simulink model "PMSM_Sinusoidal"  (R2023a)
settings: Solver=ode23t  StartTime=0.0  StopTime=5e-3  MaxStep=5e-8  RelTol=1e-5
libraries: fl_lib x4, SLSS x4, simulink_extras x1, PMSM x1, nesl_utility x1
settings Model: Creator=Szalay  LastModifiedBy=Szalay
settings SolverCC: AlgebraicLoopSolver=TrustRegion
settings DebuggingCC: UnconnectedInputMsg=warning  UnconnectedOutputMsg=warning  UnconnectedLineMsg=warning
settings ModelReferenceCC: EnableRefExpFcnMdlSchedulingChecks=on
settings RTWCC: DLArmComputeVersion=19.05
settings SimscapeCC: SimscapeLogType=all  SimscapeLogLimitData=off

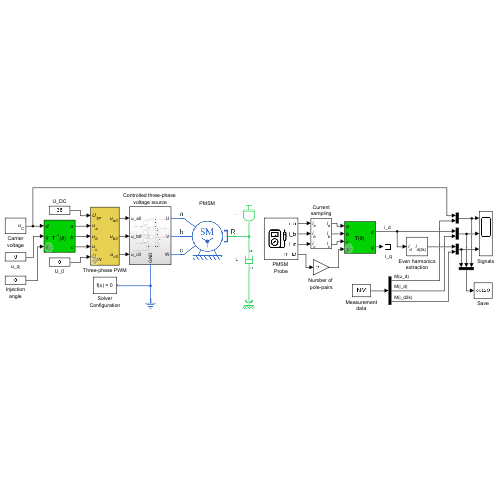
[thumbnail: Simulink's stored preview of the top-level diagram]
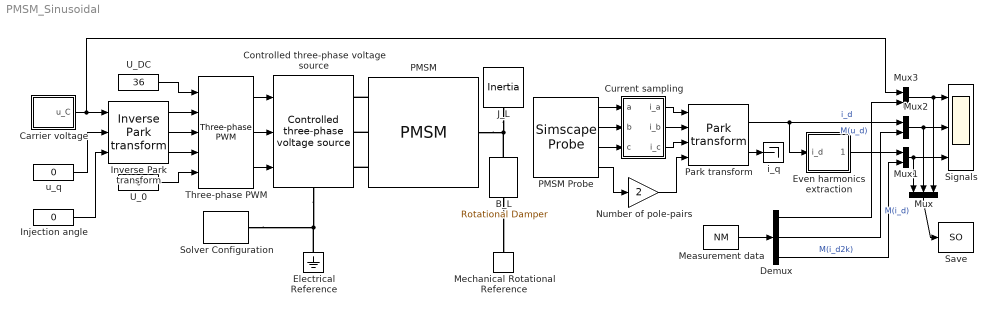
== system PMSM_Sinusoidal ==
  B_L : fl_lib/Mechanical/Rotational Elements/Rotational Damper  D=0.001 N*m*s/rad  w_specify=off  w_priority=None  w=0 rad/s  w_nominal_specify=off  w_nominal_unit=rad/s  w_nominal_value=1  t_specify=off  t_priority=None  t=0 N*m  t_nominal_specify=off  t_nominal_unit=N*m  t_nominal_value=1
  Carrier voltage : Subsystem
      mask Display: port_label('output', 1, '\itu_C', 'texmode', 'on');
  Controlled three-phase voltage source : SLSS/Power electronics/Controlled three-phase voltage source  SystemSampleTime=-1  VariantActivationTime=update diagram  Latency=0  AutoFrameSizeCalculation=off
      settings: PortSchema="{\"entries\":[{\"content\":{\"sides\":[{\"content\":{\"connectorIds\":[\"In1\",\"In2\",\"In3\"]},\"type\":\"ConnectorPlacement.EquallySpacedRectSide\",\"uuid\":\"86f4b7c9-b4c1-4fa9-92c9-df14c018ab5a\"},{\"content\":{\"connectorIds\":[\"RConn1\",\"RConn2\",\"RConn3\"],\"side\":\"RIGHT\"},\"type\":\"ConnectorPlacement.EquallySpacedRectSide\",\"uuid\":\"262f16fa-1458-4a6c-a6cd-e957fd1dcf99\"},{\"content\":{\"side\":\"TOP\"},\"type\":\"ConnectorPlacement.EquallySpacedRectSide\",\"uuid\":\"0209afef-5535-4f88-847d-86e3dc9013d0\"},{\"content\":{\"connectorIds\":[\"RConn4\"],\"side\":\"BOTTOM\"},\"type\":\"ConnectorPlacement.EquallySpacedRectSide\",\"uuid\":\"6ee3303f-0ef7-4fac-9be7-421fc8645ecd\"}]},\"type\":\"ConnectorPlacement.EquallySpacedConnector\",\"uuid\":\"dcf2ee2c-2e64-45ce-a4a6-bf45ae3145fa\"}],\"packageUris\":[\"http://schema.mathworks.com/mf0/Connector/R2020b\"],\"version\":\"1.0\"}"
  Current sampling : Subsystem
      mask Display:
      | port_label('input', 1, '\iti_a', 'texmode', 'on');
      | port_label('input', 2, '\iti_b', 'texmode', 'on');
      | port_label('input', 3, '\iti_c', 'texmode', 'on');
      | 
      | port_label('output', 1, '\iti_a', 'texmode', 'on');
      | port_label('output', 2, '\iti_b', 'texmode', 'on');
      | port_label('output', 3, '\iti_c', 'texmode', 'on');
  Demux : Demux  Outputs=3
  Electrical Reference : fl_lib/Electrical/Electrical Elements/Electrical Reference
  Even harmonics extraction : Subsystem
      mask Display:
      | port_label('input', 1, '\iti_d', 'texmode', 'on');
      | 
      | port_label('output', 1, '{\iti}_{{\itd} (2k)}', 'texmode', 'on');
  Injection angle : Constant  Value=0
  Inverse Park transform : SLSS/Transformations/Inverse Park transform  cbZero=off
  J_L : fl_lib/Mechanical/Rotational Elements/Inertia  inertia=0.0001 kg*m^2  num_ports=foundation.enum.numPorts2.one  w_specify=off  w_priority=High  w=0 rad/s  w_nominal_specify=off  w_nominal_unit=rad/s  w_nominal_value=1  t_specify=off  t_priority=None  t=0 N*m  t_nominal_specify=off  t_nominal_unit=N*m  t_nominal_value=1
  Measurement data : FromWorkspace  VariableName=NM  SampleTime=1/240000  Interpolate=off  OutputAfterFinalValue=Cyclic repetition
  Mechanical Rotational Reference : fl_lib/Mechanical/Rotational Elements/Mechanical Rotational Reference
  Mux : Mux  Inputs=3
  Mux1 : Mux  Inputs=2
  Mux2 : Mux  Inputs=2
  Mux3 : Mux  Inputs=2
  Number of pole-pairs : Gain  Gain=2
  PMSM : PMSM/PMSM  R=0.55 Ohm  z_P=2  Psi_PM=0.02483 Wb  L_dd=158e-6 H  L_qq=182e-6 H  Gamma_0=0.125e-6 H/A  J=2e-7 kg*m^2  B=6.329e-3 N*m*s/rad  th_M0=0 rad  u_a_specify=off  u_a_priority=None  u_a=0 V  u_a_nominal_specify=off  u_a_nominal_unit=V  u_a_nominal_value=1  u_b_specify=off  u_b_priority=None  u_b=0 V  u_b_nominal_specify=off  u_b_nominal_unit=V  u_b_nominal_value=1  u_c_specify=off  u_c_priority=None  u_c=0 V  u_c_nominal_specify=off  u_c_nominal_unit=V  u_c_nominal_value=1  i_a_specify=off  i_a_priority=None  i_a=0 A  i_a_nominal_specify=off  i_a_nominal_unit=A  i_a_nominal_value=1  i_b_specify=off  i_b_priority=None  i_b=0 A  i_b_nominal_specify=off  i_b_nominal_unit=A  i_b_nominal_value=1  i_c_specify=off  i_c_priority=None  i_c=0 A  i_c_nominal_specify=off  i_c_nominal_unit=A  i_c_nominal_value=1  i_n_specify=off  i_n_priority=None  i_n=0 A  i_n_nominal_specify=off  i_n_nominal_unit=A  i_n_nominal_value=1  Psi_d_specify=off  Psi_d_priority=None  Psi_d=0 Wb  Psi_d_nominal_specify=off  Psi_d_nominal_unit=Wb  Psi_d_nominal_value=1  Psi_q_specify=off  Psi_q_priority=None  Psi_q=0 Wb  Psi_q_nominal_specify=off  Psi_q_nominal_unit=Wb  Psi_q_nominal_value=1  u_d_specify=off  u_d_priority=None  u_d=0 V  u_d_nominal_specify=off  u_d_nominal_unit=V  u_d_nominal_value=1  u_q_specify=off  u_q_priority=None  u_q=0 V  u_q_nominal_specify=off  u_q_nominal_unit=V  u_q_nominal_value=1  i_d_specify=off  i_d_priority=High  i_d=0 A  i_d_nominal_specify=off  i_d_nominal_unit=A  i_d_nominal_value=1  i_q_specify=off  i_q_priority=High  i_q=0 A  i_q_nominal_specify=off  i_q_nominal_unit=A  i_q_nominal_value=1  M_E_specify=off  M_E_priority=None  M_E=0 N*m  M_E_nominal_specify=off  M_E_nominal_unit=N*m  M_E_nominal_value=1  M_L_specify=off  M_L_priority=None  M_L=0 N*m  M_L_nominal_specify=off  M_L_nominal_unit=N*m  M_L_nominal_value=1  w_M_specify=off  w_M_priority=None  w_M=0 rad/s  w_M_nominal_specify=off  w_M_nominal_unit=rad/s  w_M_nominal_value=1  w_specify=off  w_priority=None  w=0 rad/s  w_nominal_specify=off  w_nominal_unit=rad/s  w_nominal_value=1
      settings: InternalSimscapePortConfiguration="{\"Bottom\":[],\"Left\":[{\"id\":\"a\",\"label\":\"a\",\"type\":\"foundation.electrical.electrical\"},{\"id\":\"b\",\"label\":\"b\",\"type\":\"foundation.electrical.electrical\"},{\"id\":\"c\",\"label\":\"c\",\"type\":\"foundation.electrical.electrical\"}],\"Right\":[{\"id\":\"S\",\"label\":\"R\",\"type\":\"foundation.mechanical.rotational.rotational\"}],\"Top\":[]}"
  PMSM Probe : SimscapeProbe  BoundBlock=368  Variables={i_a, i_b, i_c, th_M}
  Park transform : SLSS/Transformations/Park transform  cbZero=off
  Save : ToWorkspace  VariableName=SO  SampleTime=1/240000
  Signals : Scope  NumInputPorts=3
  Solver Configuration : nesl_utility/Solver Configuration  PhysicalDomain=network_engine_domain  SubClassName=solver  LeftPortType=input  RightPortType=generic  Tones=[]  Harmonics=[]  SimulateNoise=off  Profile=off  UseLocalSampling=off  EnableSwitchedLinearOptims=on  FrequencyDomain=off  UseCCode=off  RelTol=0.001  AbsTol=0.001  MinStep=1e-09  ToWorkspace=off  RevertToSquareIcSolve=off  NumHomotopyIterations=100  PhasorMode=off  PhasorModeNumHarmonics=1  ConsistencySolver=NEWTON_XTOL_AFTER_FTOL  IndexReductionMethod=DerivativeReplacement  DoDC=on  ResidualTolerance=1e-09  ConsistencyTolSource=GLOBAL  ConsistencyAbsTol=0.001  ConsistencyRelTol=0.001  ConsistencyTolFactor=0.001  UseLocalSolver=off  LocalSolverChoice=NE_BACKWARD_EULER_ADVANCER  ResolveIndetEquations=on  FunctionEvalNumThread=1  LocalSolverSampleTime=0.001  DoFixedCost=off  MaxNonlinIter=3  MaxModeIter=2  ComputeImpulses=off  ImpulseIterations=2  LinearAlgebra=auto  LinearAlgebraNumThread=0  EquationFormulation=NE_TIME_EF  DelaysMemoryBudget=1024  AutomaticFiltering=on  FilteringTimeConstant=0.001  PartitionStorageMethod=AS_NEEDED  PartitionMemoryBudget=1024  PartitionMethod=ROBUST
  Three-phase PWM : SLSS/Power electronics/Three-phase PWM  f=40000
  U_0 : Constant  Value=0
  U_DC : Constant  Value=36
  i_q : Terminator
  u_q : Constant  Value=0
  wires:
  Inverse Park transform/1 -> Three-phase PWM/2
  U_0/1 -> Three-phase PWM/5
  U_DC/1 -> Three-phase PWM/1
  Inverse Park transform/2 -> Three-phase PWM/3
  Inverse Park transform/3 -> Three-phase PWM/4
  Number of pole-pairs/1 -> Park transform/4
  u_q/1 -> Inverse Park transform/2
  Park transform/1 -> Mux2/1, Even harmonics extraction/1(i_d)  "i_d"
  Measurement data/1 -> Demux/1
  Demux/3 -> Mux1/2  "M(i_d2k)"
  Mux2/1 -> Mux/2, Signals/2
  Demux/2 -> Mux2/2  "M(i_d)"
  Mux1/1 -> Mux/1, Signals/3
  Demux/1 -> Mux3/2  "M(u_d)"
  Carrier voltage/1(u_C) -> Inverse Park transform/1, Mux3/1
  Mux3/1 -> Mux/3, Signals/1
  PMSM Probe/1 -> Current sampling/1(a)
  PMSM Probe/2 -> Current sampling/2(b)
  PMSM Probe/3 -> Current sampling/3(c)
  Current sampling/1(i_a) -> Park transform/1
  Current sampling/2(i_b) -> Park transform/2
  Current sampling/3(i_c) -> Park transform/3
  Even harmonics extraction/1(i_d2) -> Mux1/1
  Mux/1 -> Save/1
  PMSM Probe/4 -> Number of pole-pairs/1
  Park transform/2 -> i_q/1
  Injection angle/1 -> Inverse Park transform/3
  Three-phase PWM/1 -> Controlled three-phase voltage source/1
  Three-phase PWM/2 -> Controlled three-phase voltage source/2
  Three-phase PWM/3 -> Controlled three-phase voltage source/3
  connections:
  Electrical Reference/LConn1 -- Controlled three-phase voltage source/RConn4 -- Solver Configuration/RConn1
  B_L/RConn1 -- Mechanical Rotational Reference/LConn1
  B_L/LConn1 -- PMSM/RConn1 -- J_L/LConn1
  PMSM/LConn1 -- Controlled three-phase voltage source/RConn1
  PMSM/LConn2 -- Controlled three-phase voltage source/RConn2
  PMSM/LConn3 -- Controlled three-phase voltage source/RConn3

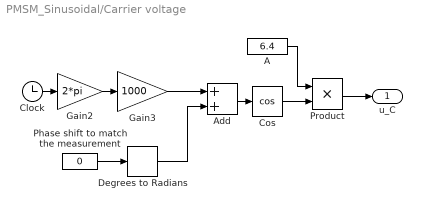
== system PMSM_Sinusoidal/Carrier voltage ==
  A : Constant  Value=6.4
  Add : Sum
  Clock : Clock
  Cos : Trigonometry  Operator=cos
  Degrees to Radians : simulink_extras/Transformations/Degrees to Radians
  Gain2 : Gain  Gain=2*pi
  Gain3 : Gain  Gain=1000
  Phase shift to match the measurement : Constant  Value=0
  Product : Product
  u_C : Outport
  wires:
  Clock/1 -> Gain2/1
  Gain2/1 -> Gain3/1
  Product/1 -> u_C/1
  Cos/1 -> Product/2
  Gain3/1 -> Add/1
  A/1 -> Product/1
  Add/1 -> Cos/1
  Phase shift to match the measurement/1 -> Degrees to Radians/1
  Degrees to Radians/1 -> Add/2

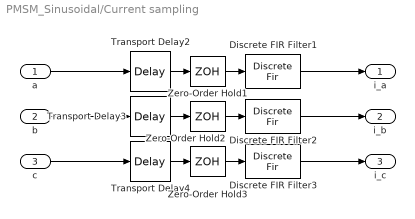
== system PMSM_Sinusoidal/Current sampling ==
  a : Inport
  b : Inport  Port=2
  c : Inport  Port=3
  Discrete FIR Filter1 : DiscreteFir  Coefficients=ones(1, 6)/6  SampleTime=1/240000
  Discrete FIR Filter2 : DiscreteFir  Coefficients=ones(1, 6)/6  SampleTime=1/240000
  Discrete FIR Filter3 : DiscreteFir  Coefficients=ones(1, 6)/6  SampleTime=1/240000
  Transport Delay2 : TransportDelay  DelayTime=1/240000/2
  Transport Delay3 : TransportDelay  DelayTime=1/240000/2
  Transport Delay4 : TransportDelay  DelayTime=1/240000/2
  Zero-Order Hold1 : ZeroOrderHold  SampleTime=1/240000
  Zero-Order Hold2 : ZeroOrderHold  SampleTime=1/240000
  Zero-Order Hold3 : ZeroOrderHold  SampleTime=1/240000
  i_a : Outport
  i_b : Outport  Port=2
  i_c : Outport  Port=3
  wires:
  Transport Delay2/1 -> Zero-Order Hold1/1
  Zero-Order Hold1/1 -> Discrete FIR Filter1/1
  Zero-Order Hold3/1 -> Discrete FIR Filter3/1
  c/1 -> Transport Delay4/1
  Zero-Order Hold2/1 -> Discrete FIR Filter2/1
  Transport Delay4/1 -> Zero-Order Hold3/1
  Transport Delay3/1 -> Zero-Order Hold2/1
  b/1 -> Transport Delay3/1
  a/1 -> Transport Delay2/1
  Discrete FIR Filter2/1 -> i_b/1
  Discrete FIR Filter1/1 -> i_a/1
  Discrete FIR Filter3/1 -> i_c/1

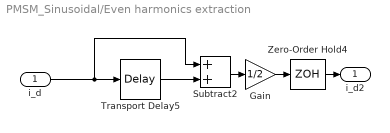
== system PMSM_Sinusoidal/Even harmonics extraction ==
  i_d : Inport
  Gain : Gain  Gain=1/2
  Subtract2 : Sum
  Transport Delay5 : TransportDelay  DelayTime=(1/240000)*240/2  BufferSize=16000
  Zero-Order Hold4 : ZeroOrderHold  SampleTime=1/240000
  i_d2 : Outport
  wires:
  Gain/1 -> Zero-Order Hold4/1
  Transport Delay5/1 -> Subtract2/2
  Subtract2/1 -> Gain/1
  Zero-Order Hold4/1 -> i_d2/1
  i_d/1 -> Transport Delay5/1, Subtract2/1
